simulink model "read_weather_data"  (Simulink 8.1)
settings: Solver=FixedStepDiscrete  StartTime=0  StopTime=8759*3600  FixedStep=3600  RelTol=1e-3
libraries: CampusEnergyModeling x1
settings Model: Creator=sfrank1  LastModifiedBy=sfrank1
settings DataIOCC: SignalLoggingSaveFormat=Dataset
settings OptimizationCC: ExpressionDepthLimit=128
settings DebuggingCC: FcnCallInpInsideContextMsg=EnableAllAsError
settings GRTTargetCC: CombineOutputUpdateFcns=on  GRTInterface=off

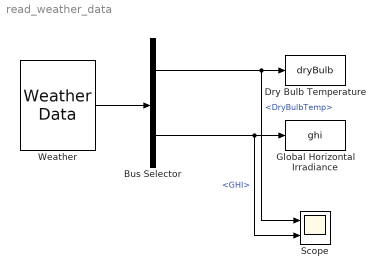
== system read_weather_data ==
  Bus Selector : BusSelector  OutputSignals=DryBulbTemp,GHI
  Dry Bulb Temperature : ToWorkspace  VariableName=dryBulb  SampleTime=-1  SaveFormat=Timeseries
  Global Horizontal Irradiance : ToWorkspace  VariableName=ghi  SampleTime=-1  SaveFormat=Timeseries
  Scope : Scope  NumInputPorts=2
      settings: ShowLegends=on  YMin=-5~-5  YMax=5~5
  Weather : CampusEnergyModeling/Weather/Weather Data  fname=weatherData.mat  initbus=on
  wires:
  Bus Selector/1 -> Scope/1, Dry Bulb Temperature/1  "<DryBulbTemp>"
  Bus Selector/2 -> Scope/2, Global Horizontal Irradiance/1  "<GHI>"
  Weather/1 -> Bus Selector/1
